simulink model "sub32_4n_model_run"  (R2023b)
settings: Solver=VariableStepAuto  StartTime=0.0  StopTime=5000E-12  FixedStep=1e-20  RelTol=1e-3
model workspace (MAT data in the model file):
  tp_delay = 1.25e-10
values from neighbouring files (symbols this model uses):
  tp_combinerA1_G8 = mean_CtoG + normrnd(0, stdev_CtoG)    [blockConf.m]
  tp_combinerA2_G4 = mean_CtoG + normrnd(0, stdev_CtoG)    [blockConf.m]
  tp_combinerA3_G2 = mean_CtoG + normrnd(0, stdev_CtoG)    [blockConf.m]
  tp_combinerA4_G1 = mean_CtoG + normrnd(0, stdev_CtoG)    [blockConf.m]
  tp_combinerB1_G8 = mean_CtoG + normrnd(0, stdev_CtoG)    [blockConf.m]
  tp_combinerB2_G4 = mean_CtoG + normrnd(0, stdev_CtoG)    [blockConf.m]
  tp_combinerB3_G2 = mean_CtoG + normrnd(0, stdev_CtoG)    [blockConf.m]
  tp_combinerB4_G1 = mean_CtoG + normrnd(0, stdev_CtoG)    [blockConf.m]
  tp_delay_1 = mean_DtoR + normrnd(0, stdev_DtoR)    [blockConf.m]
  tp_delay_10 = mean_DtoR + normrnd(0, stdev_DtoR)    [blockConf.m]
  tp_delay_11 = mean_DtoR + normrnd(0, stdev_DtoR)    [blockConf.m]
  tp_delay_12 = mean_DtoR + normrnd(0, stdev_DtoR)    [blockConf.m]
  tp_delay_13 = mean_DtoR + normrnd(0, stdev_DtoR)    [blockConf.m]
  tp_delay_14 = mean_DtoR + normrnd(0, stdev_DtoR)    [blockConf.m]
  tp_delay_15 = mean_DtoR + normrnd(0, stdev_DtoR)    [blockConf.m]
  tp_delay_16 = mean_DtoR + normrnd(0, stdev_DtoR)    [blockConf.m]
  tp_delay_17 = mean_DtoR + normrnd(0, stdev_DtoR)    [blockConf.m]
  tp_delay_18 = mean_DtoR + normrnd(0, stdev_DtoR)    [blockConf.m]
  tp_delay_19 = mean_DtoR + normrnd(0, stdev_DtoR)    [blockConf.m]
  tp_delay_2 = mean_DtoR + normrnd(0, stdev_DtoR)    [blockConf.m]
  tp_delay_20 = mean_DtoR + normrnd(0, stdev_DtoR)    [blockConf.m]
  tp_delay_21 = mean_DtoR + normrnd(0, stdev_DtoR)    [blockConf.m]
  tp_delay_22 = mean_DtoR + normrnd(0, stdev_DtoR)    [blockConf.m]
  tp_delay_23 = mean_DtoR + normrnd(0, stdev_DtoR)    [blockConf.m]
  tp_delay_24 = mean_DtoR + normrnd(0, stdev_DtoR)    [blockConf.m]
  tp_delay_25 = mean_DtoR + normrnd(0, stdev_DtoR)    [blockConf.m]
  tp_delay_26 = mean_DtoR + normrnd(0, stdev_DtoR)    [blockConf.m]
  tp_delay_27 = mean_DtoR + normrnd(0, stdev_DtoR)    [blockConf.m]
  tp_delay_28 = mean_DtoR + normrnd(0, stdev_DtoR)    [blockConf.m]
  tp_delay_29 = mean_DtoR + normrnd(0, stdev_DtoR)    [blockConf.m]
  tp_delay_3 = mean_DtoR + normrnd(0, stdev_DtoR)    [blockConf.m]
  tp_delay_30 = mean_DtoR + normrnd(0, stdev_DtoR)    [blockConf.m]
  tp_delay_31 = mean_DtoR + normrnd(0, stdev_DtoR)    [blockConf.m]
  tp_delay_32 = mean_DtoR + normrnd(0, stdev_DtoR)    [blockConf.m]
  tp_delay_4 = mean_DtoR + normrnd(0, stdev_DtoR)    [blockConf.m]
  tp_delay_5 = mean_DtoR + normrnd(0, stdev_DtoR)    [blockConf.m]
  tp_delay_6 = mean_DtoR + normrnd(0, stdev_DtoR)    [blockConf.m]
  tp_delay_7 = mean_DtoR + normrnd(0, stdev_DtoR)    [blockConf.m]
  tp_delay_8 = mean_DtoR + normrnd(0, stdev_DtoR)    [blockConf.m]
  tp_delay_9 = mean_DtoR + normrnd(0, stdev_DtoR)    [blockConf.m]
  tp_delay_b1 = mean_delay + normrnd(0, stdev_delay)    [blockConf.m]
  tp_delay_b10 = mean_delay + normrnd(0, stdev_delay)    [blockConf.m]
  tp_delay_b11 = mean_delay + normrnd(0, stdev_delay)    [blockConf.m]
  tp_delay_b12 = mean_delay + normrnd(0, stdev_delay)    [blockConf.m]
  tp_delay_b13 = mean_delay + normrnd(0, stdev_delay)    [blockConf.m]
  tp_delay_b14 = mean_delay + normrnd(0, stdev_delay)    [blockConf.m]
  tp_delay_b15 = mean_delay + normrnd(0, stdev_delay)    [blockConf.m]
  tp_delay_b16 = mean_delay + normrnd(0, stdev_delay)    [blockConf.m]
  tp_delay_b17 = mean_delay + normrnd(0, stdev_delay)    [blockConf.m]
  tp_delay_b18 = mean_delay + normrnd(0, stdev_delay)    [blockConf.m]
  tp_delay_b19 = mean_delay + normrnd(0, stdev_delay)    [blockConf.m]
  tp_delay_b2 = mean_delay + normrnd(0, stdev_delay)    [blockConf.m]
  tp_delay_b20 = mean_delay + normrnd(0, stdev_delay)    [blockConf.m]
  tp_delay_b21 = mean_delay + normrnd(0, stdev_delay)    [blockConf.m]
  tp_delay_b22 = mean_delay + normrnd(0, stdev_delay)    [blockConf.m]
  tp_delay_b23 = mean_delay + normrnd(0, stdev_delay)    [blockConf.m]
  tp_delay_b24 = mean_delay + normrnd(0, stdev_delay)    [blockConf.m]
  tp_delay_b25 = mean_delay + normrnd(0, stdev_delay)    [blockConf.m]
  tp_delay_b26 = mean_delay + normrnd(0, stdev_delay)    [blockConf.m]
  tp_delay_b27 = mean_delay + normrnd(0, stdev_delay)    [blockConf.m]
  tp_delay_b28 = mean_delay + normrnd(0, stdev_delay)    [blockConf.m]
  tp_delay_b29 = mean_delay + normrnd(0, stdev_delay)    [blockConf.m]
  tp_delay_b3 = mean_delay + normrnd(0, stdev_delay)    [blockConf.m]
  tp_delay_b30 = mean_delay + normrnd(0, stdev_delay)    [blockConf.m]
  tp_delay_b31 = mean_delay + normrnd(0, stdev_delay)    [blockConf.m]
  tp_delay_b4 = mean_delay + normrnd(0, stdev_delay)    [blockConf.m]
  tp_delay_b5 = mean_delay + normrnd(0, stdev_delay)    [blockConf.m]
  tp_delay_b6 = mean_delay + normrnd(0, stdev_delay)    [blockConf.m]
  tp_delay_b7 = mean_delay + normrnd(0, stdev_delay)    [blockConf.m]
  tp_delay_b8 = mean_delay + normrnd(0, stdev_delay)    [blockConf.m]
  tp_delay_b9 = mean_delay + normrnd(0, stdev_delay)    [blockConf.m]
  tp_pa_1 = mean_GtoP + normrnd(0, stdev_GtoP1)    [blockConf.m]
  tp_pa_2 = mean_GtoP + normrnd(0, stdev_GtoP2)    [blockConf.m]
  tp_pa_3 = mean_GtoP + normrnd(0, stdev_GtoP3)    [blockConf.m]
  tp_pa_4 = mean_GtoP + normrnd(0, stdev_GtoP4)    [blockConf.m]
  tp_router10_1 = mean_RtoC + normrnd(0, stdev_RtoC)    [blockConf.m]
  tp_router10_2 = mean_RtoC + normrnd(0, stdev_RtoC)    [blockConf.m]
  tp_router10_4 = mean_RtoC + normrnd(0, stdev_RtoC)    [blockConf.m]
  tp_router10_8 = mean_RtoC + normrnd(0, stdev_RtoC)    [blockConf.m]
  tp_router11_1 = mean_RtoC + normrnd(0, stdev_RtoC)    [blockConf.m]
  tp_router11_2 = mean_RtoC + normrnd(0, stdev_RtoC)    [blockConf.m]
  tp_router11_4 = mean_RtoC + normrnd(0, stdev_RtoC)    [blockConf.m]
  tp_router11_8 = mean_RtoC + normrnd(0, stdev_RtoC)    [blockConf.m]
  tp_router12_1 = mean_RtoC + normrnd(0, stdev_RtoC)    [blockConf.m]
  tp_router12_2 = mean_RtoC + normrnd(0, stdev_RtoC)    [blockConf.m]
  tp_router12_4 = mean_RtoC + normrnd(0, stdev_RtoC)    [blockConf.m]
  tp_router12_8 = mean_RtoC + normrnd(0, stdev_RtoC)    [blockConf.m]
  tp_router13_1 = mean_RtoC + normrnd(0, stdev_RtoC)    [blockConf.m]
  tp_router13_2 = mean_RtoC + normrnd(0, stdev_RtoC)    [blockConf.m]
  tp_router13_4 = mean_RtoC + normrnd(0, stdev_RtoC)    [blockConf.m]
  tp_router13_8 = mean_RtoC + normrnd(0, stdev_RtoC)    [blockConf.m]
  tp_router14_1 = mean_RtoC + normrnd(0, stdev_RtoC)    [blockConf.m]
  tp_router14_2 = mean_RtoC + normrnd(0, stdev_RtoC)    [blockConf.m]
  tp_router14_4 = mean_RtoC + normrnd(0, stdev_RtoC)    [blockConf.m]
  tp_router14_8 = mean_RtoC + normrnd(0, stdev_RtoC)    [blockConf.m]
  tp_router15_1 = mean_RtoC + normrnd(0, stdev_RtoC)    [blockConf.m]
  tp_router15_2 = mean_RtoC + normrnd(0, stdev_RtoC)    [blockConf.m]
  tp_router15_4 = mean_RtoC + normrnd(0, stdev_RtoC)    [blockConf.m]
  tp_router15_8 = mean_RtoC + normrnd(0, stdev_RtoC)    [blockConf.m]
  tp_router16_1 = mean_RtoC + normrnd(0, stdev_RtoC)    [blockConf.m]
  tp_router16_2 = mean_RtoC + normrnd(0, stdev_RtoC)    [blockConf.m]
  tp_router16_4 = mean_RtoC + normrnd(0, stdev_RtoC)    [blockConf.m]
  tp_router16_8 = mean_RtoC + normrnd(0, stdev_RtoC)    [blockConf.m]
  tp_router17_1 = mean_RtoC + normrnd(0, stdev_RtoC)    [blockConf.m]
  tp_router17_2 = mean_RtoC + normrnd(0, stdev_RtoC)    [blockConf.m]
  tp_router17_4 = mean_RtoC + normrnd(0, stdev_RtoC)    [blockConf.m]
  tp_router17_8 = mean_RtoC + normrnd(0, stdev_RtoC)    [blockConf.m]
  tp_router18_1 = mean_RtoC + normrnd(0, stdev_RtoC)    [blockConf.m]
  tp_router18_2 = mean_RtoC + normrnd(0, stdev_RtoC)    [blockConf.m]
  tp_router18_4 = mean_RtoC + normrnd(0, stdev_RtoC)    [blockConf.m]
  tp_router18_8 = mean_RtoC + normrnd(0, stdev_RtoC)    [blockConf.m]
  tp_router19_1 = mean_RtoC + normrnd(0, stdev_RtoC)    [blockConf.m]
  tp_router19_2 = mean_RtoC + normrnd(0, stdev_RtoC)    [blockConf.m]
  tp_router19_4 = mean_RtoC + normrnd(0, stdev_RtoC)    [blockConf.m]
  tp_router19_8 = mean_RtoC + normrnd(0, stdev_RtoC)    [blockConf.m]
  tp_router1_1 = mean_RtoC + normrnd(0, stdev_RtoC)    [blockConf.m]
  tp_router1_2 = mean_RtoC + normrnd(0, stdev_RtoC)    [blockConf.m]
  tp_router1_4 = mean_RtoC + normrnd(0, stdev_RtoC)    [blockConf.m]
  tp_router1_8 = mean_RtoC + normrnd(0, stdev_RtoC)    [blockConf.m]
  tp_router20_1 = mean_RtoC + normrnd(0, stdev_RtoC)    [blockConf.m]
  ... (+83 more)
undefined symbols (not defined in the file or in its folder): r10_1, r10_2, r10_4, r10_8, r11_1, r11_2, r11_4, r11_8, r12_1, r12_2, r12_4, r12_8, r13_1, r13_2, r13_4, r13_8, r14_1, r14_2, r14_4, r14_8, r15_1, r15_2, r15_4, r15_8, r16_1, r16_2, r16_4, r16_8, r1_1, r1_2, r1_4, r1_8, r2_1, r2_2, r2_4, r2_8, r3_1, r3_2, r3_4, r3_8, r4_1, r4_2, r4_4, r4_8, r5_1, r5_2, r5_4, r5_8, r6_1, r6_2, r6_4, r6_8, r7_1, r7_2, r7_4, r7_8, r8_1, r8_2, r8_4, r8_8 ... (+4)
libraries: fl_lib x15, nesl_utility x3, simulink x2
(part 1 of 2)
settings Model: PacingRate=0.010000  Creator=emman  LastModifiedBy=emman
settings SolverCC: EnableFixedStepZeroCrossing=on
settings OptimizationCC: ReuseModelBlockBuffer=off
settings DebuggingCC: SigSpecEnsureSampleTimeMsg=none

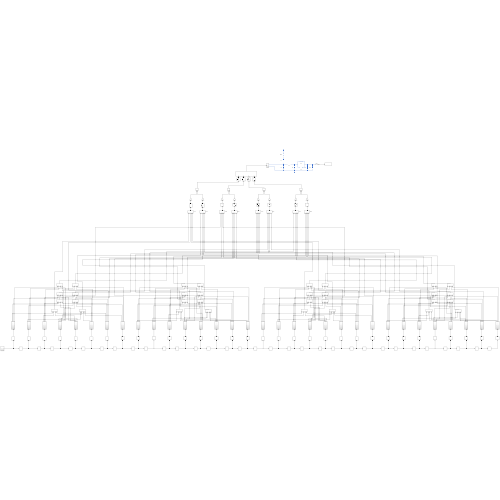
[thumbnail: Simulink's stored preview of the top-level diagram]
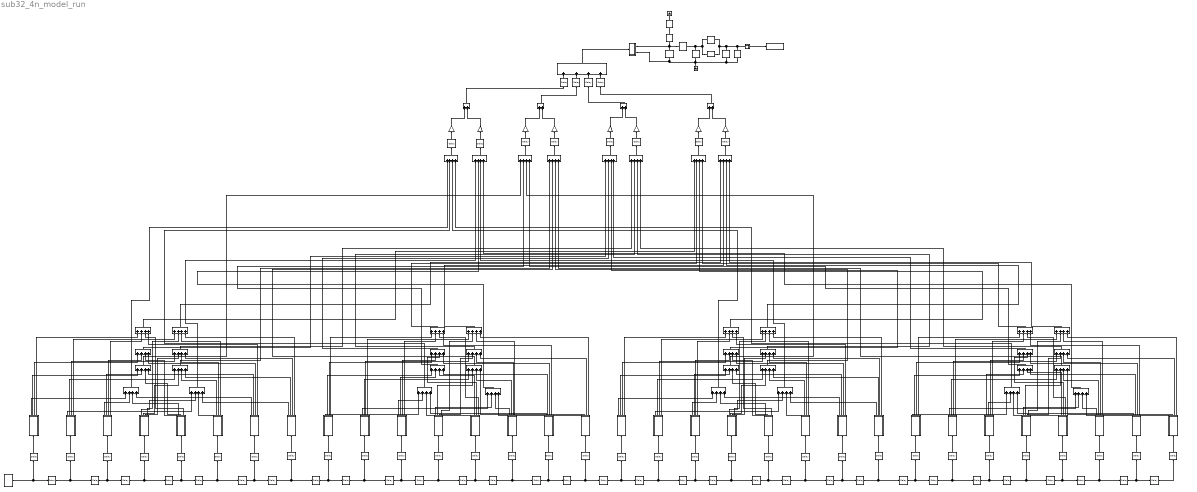
== system sub32_4n_model_run ==
  A<1> : Sum  Inputs=++++
  A<2> : Sum  Inputs=++++
  A<3> : Sum  Inputs=++++
  A<4> : Sum  Inputs=++++
  Add{,1..15,20..36} (33 alike) : Sum  Inputs=++++
  Add{16..19} (4 alike) : Sum
  B<1> : Sum  Inputs=++++
  B<2> : Sum  Inputs=++++
  B<3> : Sum  Inputs=++++
  B<4> : Sum  Inputs=++++
  C1 : fl_lib/Electrical/Electrical Elements/Capacitor  c=870e-15 F  r=0 Ohm  g=0 1/Ohm  i_specify=off  i_priority=None  i=0 A  i_nominal_specify=off  i_nominal_unit=A  i_nominal_value=1  v_specify=off  v_priority=None  v=0 V  v_nominal_specify=off  v_nominal_unit=V  v_nominal_value=1  vc_specify=off  vc_priority=High  vc=0 V  vc_nominal_specify=off  vc_nominal_unit=V  vc_nominal_value=1
  C2 : fl_lib/Electrical/Electrical Elements/Capacitor  c=1.1e-12 F  r=0 Ohm  g=0 1/Ohm  i_specify=off  i_priority=None  i=0 A  i_nominal_specify=off  i_nominal_unit=A  i_nominal_value=1  v_specify=off  v_priority=None  v=0 V  v_nominal_specify=off  v_nominal_unit=V  v_nominal_value=1  vc_specify=off  vc_priority=High  vc=0 V  vc_nominal_specify=off  vc_nominal_unit=V  vc_nominal_value=1
  C3 : fl_lib/Electrical/Electrical Elements/Capacitor  c=150e-15 F  r=0 Ohm  g=0 1/Ohm  i_specify=off  i_priority=None  i=0 A  i_nominal_specify=off  i_nominal_unit=A  i_nominal_value=1  v_specify=off  v_priority=None  v=0 V  v_nominal_specify=off  v_nominal_unit=V  v_nominal_value=1  vc_specify=off  vc_priority=High  vc=0 V  vc_nominal_specify=off  vc_nominal_unit=V  vc_nominal_value=1
  C4 : fl_lib/Electrical/Electrical Elements/Capacitor  c=70e-15 F  r=0 Ohm  g=0 1/Ohm  i_specify=off  i_priority=None  i=0 A  i_nominal_specify=off  i_nominal_unit=A  i_nominal_value=1  v_specify=off  v_priority=None  v=0 V  v_nominal_specify=off  v_nominal_unit=V  v_nominal_value=1  vc_specify=off  vc_priority=High  vc=0 V  vc_nominal_specify=off  vc_nominal_unit=V  vc_nominal_value=1
  C5 : fl_lib/Electrical/Electrical Elements/Capacitor  c=410e-15 F  r=0 Ohm  g=0 1/Ohm  i_specify=off  i_priority=None  i=0 A  i_nominal_specify=off  i_nominal_unit=A  i_nominal_value=1  v_specify=off  v_priority=None  v=0 V  v_nominal_specify=off  v_nominal_unit=V  v_nominal_value=1  vc_specify=off  vc_priority=High  vc=0 V  vc_nominal_specify=off  vc_nominal_unit=V  vc_nominal_value=1
  Current Source : Subsystem
  Electrical Reference : fl_lib/Electrical/Electrical Elements/Electrical Reference
  Electrical Reference1 : fl_lib/Electrical/Electrical Elements/Electrical Reference
  Gain : Gain  Gain=8
  Gain1 : Gain  Gain=8
  Gain2 : Gain  Gain=4
  Gain3 : Gain  Gain=4
  Gain4 : Gain  Gain=2
  Gain5 : Gain  Gain=2
  Gain6 : Gain
  Gain7 : Gain
  L1 : fl_lib/Electrical/Electrical Elements/Inductor  l=420e-12 H  r=0 Ohm  g=0 1/Ohm  i_specify=off  i_priority=None  i=0 A  i_nominal_specify=off  i_nominal_unit=A  i_nominal_value=1  v_specify=off  v_priority=None  v=0 V  v_nominal_specify=off  v_nominal_unit=V  v_nominal_value=1  i_L_specify=off  i_L_priority=High  i_L=0 A  i_L_nominal_specify=off  i_L_nominal_unit=A  i_L_nominal_value=1
  L2 : fl_lib/Electrical/Electrical Elements/Inductor  l=820e-12 H  r=0 Ohm  g=0 1/Ohm  i_specify=off  i_priority=None  i=0 A  i_nominal_specify=off  i_nominal_unit=A  i_nominal_value=1  v_specify=off  v_priority=None  v=0 V  v_nominal_specify=off  v_nominal_unit=V  v_nominal_value=1  i_L_specify=off  i_L_priority=High  i_L=0 A  i_L_nominal_specify=off  i_L_nominal_unit=A  i_L_nominal_value=1
  R0 : fl_lib/Electrical/Electrical Elements/Resistor  R=50 Ohm  i_specify=off  i_priority=None  i=0 A  i_nominal_specify=off  i_nominal_unit=A  i_nominal_value=1  v_specify=off  v_priority=None  v=0 V  v_nominal_specify=off  v_nominal_unit=V  v_nominal_value=1
  Simscape : Subsystem
      mask Display: disp('V')
  Subsystem : Subsystem
  Subsystem1 : Subsystem
  Subsystem10 : Subsystem
  Subsystem11 : Subsystem
  Subsystem12 : Subsystem
  Subsystem13 : Subsystem
  Subsystem14 : Subsystem
  Subsystem15 : Subsystem
  Subsystem16 : Subsystem
  Subsystem17 : Subsystem
  Subsystem18 : Subsystem
  Subsystem19 : Subsystem
  Subsystem2 : Subsystem
  Subsystem20 : Subsystem
  Subsystem21 : Subsystem
  Subsystem22 : Subsystem
  Subsystem23 : Subsystem
  Subsystem24 : Subsystem
  Subsystem25 : Subsystem
  Subsystem26 : Subsystem
  Subsystem27 : Subsystem
  Subsystem28 : Subsystem
  Subsystem29 : Subsystem
  Subsystem3 : Subsystem
  Subsystem30 : Subsystem
  Subsystem31 : Subsystem
  Subsystem32 : Subsystem
  Subsystem4 : Subsystem
  Subsystem5 : Subsystem
  Subsystem6 : Subsystem
  Subsystem7 : Subsystem
  Subsystem8 : Subsystem
  Subsystem9 : Subsystem
  To Workspace : ToWorkspace  VariableName=gpulse  SaveFormat=Timeseries  SampleTime=10e-12
  Transport Delay : TransportDelay  DelayTime=tp_delay_b1
  Transport Delay1 : TransportDelay  DelayTime=tp_delay_b2
  Transport Delay10 : TransportDelay  DelayTime=tp_delay_b11
  Transport Delay101 : TransportDelay  DelayTime=tp_delay_b22
  Transport Delay102 : TransportDelay  DelayTime=tp_delay_b23
  Transport Delay103 : TransportDelay  DelayTime=tp_delay_b24
  Transport Delay104 : TransportDelay  DelayTime=tp_delay_b25
  Transport Delay105 : TransportDelay  DelayTime=tp_delay_b26
  Transport Delay106 : TransportDelay  DelayTime=tp_delay_b16
  Transport Delay11 : TransportDelay  DelayTime=tp_delay_b12
  Transport Delay12 : TransportDelay  DelayTime=tp_delay_b13
  Transport Delay13 : TransportDelay  DelayTime=tp_delay_b14
  Transport Delay14 : TransportDelay  DelayTime=tp_delay_b15
  Transport Delay15 : TransportDelay  DelayTime=tp_delay_1
  Transport Delay16 : TransportDelay  DelayTime=tp_delay_2
  Transport Delay17 : TransportDelay  DelayTime=tp_delay_3
  Transport Delay18 : TransportDelay  DelayTime=tp_delay_4
  Transport Delay19 : TransportDelay  DelayTime=tp_delay_5
  Transport Delay2 : TransportDelay  DelayTime=tp_delay_b3
  Transport Delay20 : TransportDelay  DelayTime=tp_delay_6
  Transport Delay21 : TransportDelay  DelayTime=tp_delay_7
  Transport Delay22 : TransportDelay  DelayTime=tp_delay_8
  Transport Delay23 : TransportDelay  DelayTime=tp_delay_9
  Transport Delay24 : TransportDelay  DelayTime=tp_delay_10
  Transport Delay25 : TransportDelay  DelayTime=tp_delay_11
  Transport Delay26 : TransportDelay  DelayTime=tp_delay_12
  Transport Delay27 : TransportDelay  DelayTime=tp_delay_13
  Transport Delay28 : TransportDelay  DelayTime=tp_delay_14
  Transport Delay29 : TransportDelay  DelayTime=tp_delay_15
  Transport Delay3 : TransportDelay  DelayTime=tp_delay_b4
  Transport Delay30 : TransportDelay  DelayTime=tp_delay_16
  Transport Delay4 : TransportDelay  DelayTime=tp_delay_b5
  Transport Delay47 : TransportDelay  DelayTime=tp_combinerA1_G8
  Transport Delay48 : TransportDelay  DelayTime=tp_combinerB1_G8
  Transport Delay49 : TransportDelay  DelayTime=tp_combinerA2_G4
  Transport Delay5 : TransportDelay  DelayTime=tp_delay_b6
  Transport Delay50 : TransportDelay  DelayTime=tp_combinerB2_G4
  Transport Delay51 : TransportDelay  DelayTime=tp_combinerA3_G2
  Transport Delay52 : TransportDelay  DelayTime=tp_combinerB3_G2
  Transport Delay53 : TransportDelay  DelayTime=tp_combinerA4_G1
  Transport Delay54 : TransportDelay  DelayTime=tp_combinerB4_G1
  Transport Delay55 : TransportDelay  DelayTime=tp_pa_1  TransDelayFeedthrough=on
  Transport Delay56 : TransportDelay  DelayTime=tp_pa_2  TransDelayFeedthrough=on
  Transport Delay57 : TransportDelay  DelayTime=tp_pa_3  TransDelayFeedthrough=on
  Transport Delay58 : TransportDelay  DelayTime=tp_pa_4  TransDelayFeedthrough=on
  Transport Delay59 : TransportDelay  DelayTime=tp_delay_b17
  Transport Delay6 : TransportDelay  DelayTime=tp_delay_b7
  Transport Delay60 : TransportDelay  DelayTime=tp_delay_b18
  Transport Delay61 : TransportDelay  DelayTime=tp_delay_b27
  Transport Delay62 : TransportDelay  DelayTime=tp_delay_b28
  Transport Delay63 : TransportDelay  DelayTime=tp_delay_b29
  Transport Delay64 : TransportDelay  DelayTime=tp_delay_b30
  Transport Delay65 : TransportDelay  DelayTime=tp_delay_b31
  Transport Delay66 : TransportDelay  DelayTime=tp_delay_17
  Transport Delay67 : TransportDelay  DelayTime=tp_delay_18
  Transport Delay68 : TransportDelay  DelayTime=tp_delay_19
  Transport Delay69 : TransportDelay  DelayTime=tp_delay_20
  Transport Delay7 : TransportDelay  DelayTime=tp_delay_b8
  Transport Delay70 : TransportDelay  DelayTime=tp_delay_21
  Transport Delay71 : TransportDelay  DelayTime=tp_delay_b19
  Transport Delay72 : TransportDelay  DelayTime=tp_delay_22
  Transport Delay73 : TransportDelay  DelayTime=tp_delay_23
  Transport Delay74 : TransportDelay  DelayTime=tp_delay_24
  Transport Delay75 : TransportDelay  DelayTime=tp_delay_25
  Transport Delay76 : TransportDelay  DelayTime=tp_delay_26
  Transport Delay77 : TransportDelay  DelayTime=tp_delay_27
  Transport Delay78 : TransportDelay  DelayTime=tp_delay_28
  Transport Delay79 : TransportDelay  DelayTime=tp_delay_29
  Transport Delay8 : TransportDelay  DelayTime=tp_delay_b9
  Transport Delay80 : TransportDelay  DelayTime=tp_delay_30
  Transport Delay81 : TransportDelay  DelayTime=tp_delay_31
  Transport Delay82 : TransportDelay  DelayTime=tp_delay_b20
  Transport Delay83 : TransportDelay  DelayTime=tp_delay_32
  Transport Delay9 : TransportDelay  DelayTime=tp_delay_b10
  Transport Delay93 : TransportDelay  DelayTime=tp_delay_b21
  VDD : fl_lib/Electrical/Electrical Sources/DC Voltage Source  v0=0.8 V
  wires:
  Subsystem16/1(Out1) -> Add/1
  Subsystem18/1(Out1) -> Add/2
  Subsystem20/1(Out1) -> Add/3
  Subsystem17/1(Out1) -> Add1/1
  Subsystem21/1(Out1) -> Add1/3
  Subsystem23/1(Out1) -> Add1/4
  Subsystem19/1(Out1) -> Add1/2
  Subsystem16/2(Out2) -> Add2/1
  Subsystem20/2(Out2) -> Add2/3
  Subsystem22/2(Out2) -> Add2/4
  Subsystem18/2(Out2) -> Add2/2
  Subsystem17/2(Out2) -> Add3/1
  Subsystem19/2(Out2) -> Add3/2
  Subsystem21/2(Out2) -> Add3/3
  Subsystem23/2(Out2) -> Add3/4
  Subsystem17/3(Out3) -> Add5/1
  Subsystem22/3(Out3) -> Add4/4
  Subsystem16/4(Out4) -> Add6/1
  Subsystem19/3(Out3) -> Add5/2
  Subsystem20/4(Out4) -> Add6/3
  Subsystem18/4(Out4) -> Add6/2
  Subsystem21/4(Out4) -> Add7/3
  Subsystem18/3(Out3) -> Add4/2
  Subsystem16/3(Out3) -> Add4/1
  Subsystem23/4(Out4) -> Add7/4
  Subsystem19/4(Out4) -> Add7/2
  Subsystem20/3(Out3) -> Add4/3
  Subsystem17/4(Out4) -> Add7/1
  Subsystem21/3(Out3) -> Add5/3
  Subsystem23/3(Out3) -> Add5/4
  Subsystem8/4(Out4) -> Add14/1
  Subsystem3/4(Out4) -> Add15/3
  Subsystem5/2(Out2) -> Add11/2
  Subsystem2/2(Out2) -> Add10/4
  Subsystem7/1(Out1) -> Add9/1
  Subsystem5/1(Out1) -> Add9/2
  Subsystem4/1(Out1) -> Add8/3
  Subsystem1/4(Out4) -> Add15/4
  Subsystem8/3(Out3) -> Add12/1
  Subsystem2/3(Out3) -> Add12/4
  Subsystem7/3(Out3) -> Add13/1
  Subsystem4/3(Out3) -> Add12/3
  Subsystem4/2(Out2) -> Add10/3
  Subsystem3/2(Out2) -> Add11/3
  Subsystem1/3(Out3) -> Add13/4
  Subsystem6/3(Out3) -> Add12/2
  Subsystem1/1(Out1) -> Add9/4
  Subsystem7/4(Out4) -> Add15/1
  Subsystem2/1(Out1) -> Add8/4
  Subsystem8/2(Out2) -> Add10/1
  Subsystem2/4(Out4) -> Add14/4
  Subsystem6/4(Out4) -> Add14/2
  Subsystem1/2(Out2) -> Add11/4
  Subsystem8/1(Out1) -> Add8/1
  Subsystem3/3(Out3) -> Add13/3
  Subsystem7/2(Out2) -> Add11/1
  Subsystem4/4(Out4) -> Add14/3
  Subsystem5/4(Out4) -> Add15/2
  Subsystem3/1(Out1) -> Add9/3
  Subsystem5/3(Out3) -> Add13/2
  Gain/1 -> Add16/1
  Gain1/1 -> Add16/2
  Gain3/1 -> Add17/2
  Gain2/1 -> Add17/1
  Gain5/1 -> Add18/2
  Gain4/1 -> Add18/1
  Gain6/1 -> Add19/1
  Gain7/1 -> Add19/2
  Add16/1 -> Transport Delay55/1
  Add17/1 -> Transport Delay56/1
  Add18/1 -> Transport Delay57/1
  Add19/1 -> Transport Delay58/1
  Add20/1 -> Current Source/1(I)
  Simscape/1(Out) -> To Workspace/1  "output"
  Transport Delay3/1 -> Transport Delay4/1, Transport Delay19/1
  Transport Delay5/1 -> Transport Delay21/1, Transport Delay6/1
  Transport Delay4/1 -> Transport Delay20/1, Transport Delay5/1
  Transport Delay6/1 -> Transport Delay22/1, Transport Delay7/1
  Transport Delay13/1 -> Transport Delay29/1, Transport Delay14/1
  Transport Delay11/1 -> Transport Delay27/1, Transport Delay12/1
  Transport Delay10/1 -> Transport Delay26/1, Transport Delay11/1
  Transport Delay8/1 -> Transport Delay24/1, Transport Delay9/1
  Transport Delay9/1 -> Transport Delay25/1, Transport Delay10/1
  Transport Delay12/1 -> Transport Delay28/1, Transport Delay13/1
  A<3>/1 -> Transport Delay51/1
  A<4>/1 -> Transport Delay53/1
  B<4>/1 -> Transport Delay54/1
  B<3>/1 -> Transport Delay52/1
  Subsystem/1(Out1) -> Transport Delay15/1, Transport Delay/1
  Transport Delay/1 -> Transport Delay16/1, Transport Delay1/1
  Transport Delay1/1 -> Transport Delay17/1, Transport Delay2/1
  A<2>/1 -> Transport Delay49/1
  B<1>/1 -> Transport Delay48/1
  Transport Delay7/1 -> Transport Delay23/1, Transport Delay8/1
  Subsystem22/4(Out4) -> Add6/4
  Subsystem22/1(Out1) -> Add/4
  A<1>/1 -> Transport Delay47/1
  B<2>/1 -> Transport Delay50/1
  Transport Delay2/1 -> Transport Delay18/1, Transport Delay3/1
  Transport Delay15/1 -> Subsystem16/1(In1)
  Transport Delay16/1 -> Subsystem17/1(In1)
  Transport Delay17/1 -> Subsystem18/1(In1)
  Transport Delay18/1 -> Subsystem19/1(In1)
  Transport Delay19/1 -> Subsystem20/1(In1)
  Transport Delay20/1 -> Subsystem21/1(In1)
  Transport Delay21/1 -> Subsystem22/1(In1)
  Transport Delay22/1 -> Subsystem23/1(In1)
  Transport Delay23/1 -> Subsystem8/1(In1)
  Transport Delay24/1 -> Subsystem7/1(In1)
  Transport Delay25/1 -> Subsystem6/1(In1)
  Transport Delay26/1 -> Subsystem5/1(In1)
  Transport Delay27/1 -> Subsystem4/1(In1)
  Transport Delay28/1 -> Subsystem3/1(In1)
  Transport Delay29/1 -> Subsystem2/1(In1)
  Transport Delay30/1 -> Subsystem1/1(In1)
  Add/1 -> A<1>/1
  Add8/1 -> A<1>/2
  Add1/1 -> B<1>/1
  Add9/1 -> B<1>/2
  Add2/1 -> A<2>/1
  Add10/1 -> A<2>/2
  Add3/1 -> B<2>/1
  Add11/1 -> B<2>/2
  Add4/1 -> A<3>/1
  Add12/1 -> A<3>/2
  Add5/1 -> B<3>/1
  Add13/1 -> B<3>/2
  Add6/1 -> A<4>/1
  Add14/1 -> A<4>/2
  Add7/1 -> B<4>/1
  Add15/1 -> B<4>/2
  Transport Delay47/1 -> Gain/1
  Transport Delay48/1 -> Gain1/1
  Transport Delay49/1 -> Gain2/1
  Transport Delay50/1 -> Gain3/1
  Transport Delay51/1 -> Gain4/1
  Transport Delay52/1 -> Gain5/1
  Transport Delay53/1 -> Gain6/1
  Transport Delay54/1 -> Gain7/1
  Transport Delay55/1 -> Add20/1
  Transport Delay56/1 -> Add20/2
  Transport Delay57/1 -> Add20/3
  Transport Delay58/1 -> Add20/4
  Subsystem14/4(Out4) -> Add27/4
  Subsystem14/1(Out1) -> Add35/4
  Subsystem30/1(Out1) -> Add23/2
  Subsystem24/3(Out3) -> Add32/3
  Subsystem10/3(Out3) -> Add31/1
  Transport Delay66/1 -> Subsystem10/1(In1)
  Transport Delay103/1 -> Transport Delay75/1, Transport Delay104/1
  Transport Delay63/1 -> Transport Delay80/1, Transport Delay64/1
  Transport Delay60/1 -> Transport Delay68/1, Transport Delay71/1
  Subsystem28/3(Out3) -> Add25/3
  Subsystem12/3(Out3) -> Add31/2
  Transport Delay82/1 -> Transport Delay93/1, Transport Delay70/1
  Subsystem13/4(Out4) -> Add34/2
  Subsystem25/3(Out3) -> Add31/4
  Transport Delay105/1 -> Transport Delay77/1, Transport Delay61/1
  Subsystem29/2(Out2) -> Add24/2
  Transport Delay62/1 -> Transport Delay79/1, Transport Delay63/1
  Add36/1 -> B<1>/4
  Subsystem27/4(Out4) -> Add28/3
  Add28/1 -> B<4>/4
  Subsystem10/1(Out1) -> Add21/1
  Subsystem25/2(Out2) -> Add29/4
  Transport Delay104/1 -> Transport Delay76/1, Transport Delay105/1
  Subsystem25/1(Out1) -> Add21/4
  Subsystem11/2(Out2) -> Add30/1
  Subsystem12/2(Out2) -> Add29/2
  Subsystem15/2(Out2) -> Add29/3
  Subsystem26/2(Out2) -> Add30/4
  Transport Delay93/1 -> Transport Delay72/1, Transport Delay101/1
  Subsystem31/1(Out1) -> Add36/1
  Transport Delay76/1 -> Subsystem31/1(In1)
  Subsystem9/1(Out1) -> Add36/4
  Transport Delay77/1 -> Subsystem30/1(In1)
  Transport Delay75/1 -> Subsystem32/1(In1)
  Subsystem32/3(Out3) -> Add25/1
  Transport Delay80/1 -> Subsystem27/1(In1)
  Subsystem27/1(Out1) -> Add36/3
  Transport Delay72/1 -> Subsystem24/1(In1)
  Transport Delay69/1 -> Subsystem13/1(In1)
  Subsystem24/2(Out2) -> Add30/3
  Transport Delay67/1 -> Subsystem11/1(In1)
  Subsystem31/3(Out3) -> Add26/1
  Transport Delay14/1 -> Transport Delay106/1, Transport Delay30/1
  Subsystem11/4(Out4) -> Add34/1
  Subsystem29/4(Out4) -> Add28/2
  Subsystem24/1(Out1) -> Add22/3
  Transport Delay70/1 -> Subsystem15/1(In1)
  Transport Delay78/1 -> Subsystem29/1(In1)
  Add31/1 -> A<3>/3
  Subsystem15/3(Out3) -> Add31/3
  Transport Delay101/1 -> Transport Delay73/1, Transport Delay102/1
  Subsystem31/4(Out4) -> Add28/1
  Transport Delay102/1 -> Transport Delay74/1, Transport Delay103/1
  Subsystem28/2(Out2) -> Add23/3
  Add23/1 -> A<2>/4
  Subsystem10/4(Out4) -> Add33/1
  Subsystem15/4(Out4) -> Add33/3
  Transport Delay79/1 -> Subsystem28/1(In1)
  Subsystem9/4(Out4) -> Add28/4
  Transport Delay83/1 -> Subsystem9/1(In1)
  Subsystem14/2(Out2) -> Add23/4
  Transport Delay59/1 -> Transport Delay67/1, Transport Delay60/1
  Subsystem26/3(Out3) -> Add32/4
  Subsystem26/4(Out4) -> Add34/4
  Subsystem12/4(Out4) -> Add33/2
  Add26/1 -> B<3>/4
  Add27/1 -> A<4>/4
  Add24/1 -> B<2>/4
  Subsystem31/2(Out2) -> Add24/1
  Subsystem15/1(Out1) -> Add21/3
  Subsystem26/1(Out1) -> Add22/4
  Subsystem30/3(Out3) -> Add25/2
  Subsystem24/4(Out4) -> Add34/3
  Subsystem28/4(Out4) -> Add27/3
  Subsystem27/2(Out2) -> Add24/3
  Transport Delay68/1 -> Subsystem12/1(In1)
  Subsystem32/4(Out4) -> Add27/1
  Transport Delay64/1 -> Transport Delay81/1, Transport Delay65/1
  Subsystem13/2(Out2) -> Add30/2
  Subsystem29/1(Out1) -> Add36/2
  Transport Delay74/1 -> Subsystem26/1(In1)
  Subsystem13/3(Out3) -> Add32/2
  Subsystem14/3(Out3) -> Add25/4
  Transport Delay73/1 -> Subsystem25/1(In1)
  Subsystem30/4(Out4) -> Add27/2
  Subsystem9/2(Out2) -> Add24/4
  Subsystem32/2(Out2) -> Add23/1
  Subsystem32/1(Out1) -> Add35/1
  Subsystem30/2(Out2) -> Add35/2
  Subsystem10/2(Out2) -> Add29/1
  Subsystem9/3(Out3) -> Add26/4
  Subsystem28/1(Out1) -> Add35/3
  Subsystem27/3(Out3) -> Add26/3
  Subsystem12/1(Out1) -> Add21/2
  Transport Delay81/1 -> Subsystem14/1(In1)
  Add25/1 -> A<3>/4
  Subsystem11/3(Out3) -> Add32/1
  Add33/1 -> A<4>/3
  Subsystem13/1(Out1) -> Add22/2
  Transport Delay65/1 -> Transport Delay83/1
  Transport Delay61/1 -> Transport Delay78/1, Transport Delay62/1
  Transport Delay71/1 -> Transport Delay69/1, Transport Delay82/1
  Add21/1 -> A<1>/3
  Add32/1 -> B<3>/3
  Add35/1 -> A<1>/4
  Add22/1 -> B<1>/3
  Subsystem11/1(Out1) -> Add22/1
  Subsystem25/4(Out4) -> Add33/4
  Add29/1 -> A<2>/3
  Subsystem29/3(Out3) -> Add26/2
  Add30/1 -> B<2>/3
  Add34/1 -> B<4>/3
  Transport Delay106/1 -> Transport Delay59/1, Transport Delay66/1
  Subsystem6/1(Out1) -> Add8/2
  Subsystem6/2(Out2) -> Add10/2
  connections:
  Electrical Reference/LConn1 -- Current Source/RConn2 -- C1/RConn1 -- R0/RConn1 -- C5/RConn1 -- C3/RConn1
  C4/RConn1 -- L2/RConn1 -- Simscape/LConn1 -- R0/LConn1 -- C5/LConn1
  L2/LConn1 -- C4/LConn1 -- C3/LConn1 -- C2/RConn1
  VDD/RConn1 -- Electrical Reference1/LConn1
  L1/LConn1 -- VDD/LConn1
  C2/LConn1 -- Current Source/RConn1 -- L1/RConn1 -- C1/LConn1

== system sub32_4n_model_run/Current Source ==
  I : Inport
  Controlled Voltage Source : fl_lib/Electrical/Electrical Sources/Controlled Voltage Source
  Simulink-PS Converter : nesl_utility/Simulink-PS Converter  PhysicalDomain=network_engine_domain  SubClassName=ps_input  LeftPortType=input  RightPortType=output  PseudoPeriodic=off  Frequencies=[]  NoiseDistribution=none  NoiseParameters=[]  Unit=1  AffineConversion=off  FilteringAndDerivatives=zero  SimscapeFilterOrder=1  InputFilterTimeConstant=.001  UdotUserProvided=0
  Solver Configuration : nesl_utility/Solver Configuration  PhysicalDomain=network_engine_domain  SubClassName=solver  LeftPortType=input  RightPortType=generic  Tones=[]  Harmonics=[]  SimulateNoise=off  Profile=off  UseLocalSampling=off  EnableSwitchedLinearOptims=on  FrequencyDomain=off  UseCCode=off  RelTol=0.001  AbsTol=1e-06  MinStep=1e-09  ToWorkspace=off  RevertToSquareIcSolve=off  NumHomotopyIterations=100  PhasorMode=off  PhasorModeNumHarmonics=1  ConsistencySolver=NEWTON_FTOL  IndexReductionMethod=DerivativeReplacement  DoDC=on  ResidualTolerance=1e-15  ConsistencyTolSource=GLOBAL  ConsistencyAbsTol=0.001  ConsistencyRelTol=0.001  ConsistencyTolFactor=0.001  UseLocalSolver=off  LocalSolverChoice=NE_TRAPEZOIDAL_ADVANCER  ResolveIndetEquations=on  FunctionEvalNumThread=1  LocalSolverSampleTime=.001  DoFixedCost=on  MaxNonlinIter=3  MaxModeIter=2  ComputeImpulses=on  ImpulseIterations=2  LinearAlgebra=Full  LinearAlgebraNumThread=0  EquationFormulation=NE_TIME_EF  DelaysMemoryBudget=1024  AutomaticFiltering=off  FilteringTimeConstant=0.001  PartitionStorageMethod=AS_NEEDED  PartitionMemoryBudget=1024  PartitionMethod=FAST  MultibodyUseLocalSolver=off  MultibodyLocalSolverChoice=ODE1  MultibodyLocalSolverSampleTime=0.001
  Voltage-Controlled Current Source : fl_lib/Electrical/Electrical Sources/Voltage-Controlled Current Source  K=10 mS  v1_specify=off  v1_priority=None  v1=0 V  v1_nominal_specify=off  v1_nominal_unit=V  v1_nominal_value=1  i2_specify=off  i2_priority=None  i2=0 A  i2_nominal_specify=off  i2_nominal_unit=A  i2_nominal_value=1
      settings: InternalSimscapePortConfiguration="{\"Bottom\":[],\"Left\":[{\"id\":\"p1\",\"label\":\"+\",\"type\":\"foundation.electrical.electrical\"},{\"id\":\"head\",\"label\":\"\",\"type\":\"foundation.electrical.electrical\"}],\"Right\":[{\"id\":\"n1\",\"label\":\"-\",\"type\":\"foundation.electrical.electrical\"},{\"id\":\"tail\",\"label\":\"\",\"type\":\"foundation.electrical.electrical\"}],\"Top\":[]}"
  + : PMIOPort  Side=Right
  - : PMIOPort  Port=2  Side=Right
  wires:
  I/1 -> Simulink-PS Converter/1
  connections:
  Simulink-PS Converter/RConn1 -- Solver Configuration/RConn1 -- Controlled Voltage Source/RConn1
  -/RConn1 -- Controlled Voltage Source/RConn2 -- Voltage-Controlled Current Source/RConn1 -- Voltage-Controlled Current Source/RConn2
  +/RConn1 -- Voltage-Controlled Current Source/LConn2
  Controlled Voltage Source/LConn1 -- Voltage-Controlled Current Source/LConn1

== system sub32_4n_model_run/Simscape ==
  Electrical Reference1 : fl_lib/Electrical/Electrical Elements/Electrical Reference
  PS-S : nesl_utility/PS-Simulink Converter  PhysicalDomain=network_engine_domain  SubClassName=ps_output  LeftPortType=input  RightPortType=output  PseudoPeriodic=off  Frequencies=[]  VectorFormat=1-D array  Unit=V  AffineConversion=off
  Voltage Sensor : fl_lib/Electrical/Electrical Sensors/Voltage Sensor
  V : PMIOPort  Side=Left
  Out : Outport  VectorParamsAs1DForOutWhenUnconnected=off
  wires:
  PS-S/1 -> Out/1  "voltage"
  connections:
  PS-S/LConn1 -- Voltage Sensor/RConn1
  V/RConn1 -- Voltage Sensor/LConn1
  Electrical Reference1/LConn1 -- Voltage Sensor/RConn2

== system sub32_4n_model_run/Subsystem ==
  Add21 : Sum
  Ramp : simulink/Sources/Ramp  slope=80e+9  start=10e-12  InitialOutput=0
  Ramp1 : simulink/Sources/Ramp  slope=-80e+9  start=72.5e-12  InitialOutput=0
  Saturation : Saturate  UpperLimit=800e-3  LowerLimit=0
  Saturation1 : Saturate  UpperLimit=0  LowerLimit=-800e-3
  Out1 : Outport
  wires:
  Ramp/1 -> Saturation/1
  Saturation/1 -> Add21/1
  Ramp1/1 -> Saturation1/1
  Saturation1/1 -> Add21/2
  Add21/1 -> Out1/1

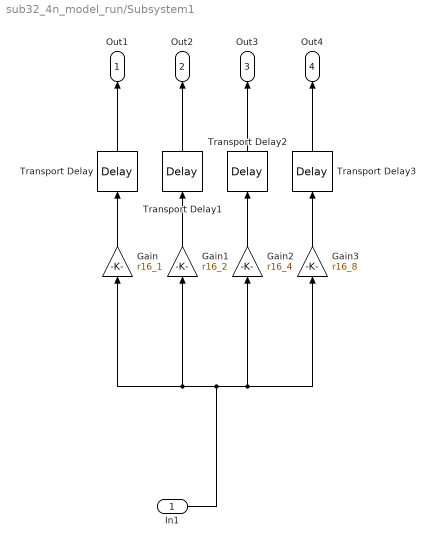
== system sub32_4n_model_run/Subsystem1 ==
  In1 : Inport
  Gain : Gain  Gain=r16_1
  Gain1 : Gain  Gain=r16_2
  Gain2 : Gain  Gain=r16_4
  Gain3 : Gain  Gain=r16_8
  Transport Delay : TransportDelay  DelayTime=tp_router16_1
  Transport Delay1 : TransportDelay  DelayTime=tp_router16_2
  Transport Delay2 : TransportDelay  DelayTime=tp_router16_4
  Transport Delay3 : TransportDelay  DelayTime=tp_router16_8
  Out1 : Outport
  Out2 : Outport  Port=2
  Out3 : Outport  Port=3
  Out4 : Outport  Port=4
  wires:
  Gain/1 -> Transport Delay/1
  Gain3/1 -> Transport Delay3/1
  Gain1/1 -> Transport Delay1/1
  In1/1 -> Gain1/1, Gain/1, Gain3/1, Gain2/1
  Gain2/1 -> Transport Delay2/1
  Transport Delay/1 -> Out1/1
  Transport Delay1/1 -> Out2/1
  Transport Delay2/1 -> Out3/1
  Transport Delay3/1 -> Out4/1

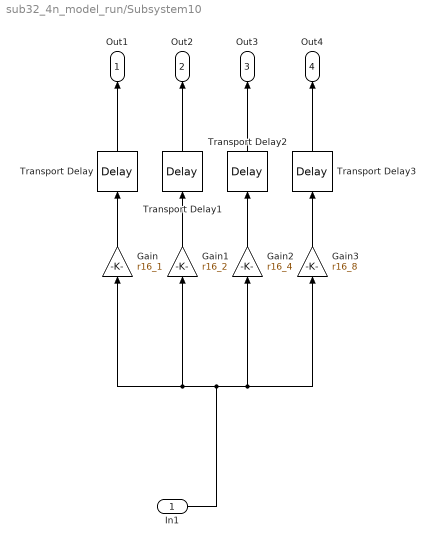
== system sub32_4n_model_run/Subsystem10 ==
  In1 : Inport
  Gain : Gain  Gain=r16_1
  Gain1 : Gain  Gain=r16_2
  Gain2 : Gain  Gain=r16_4
  Gain3 : Gain  Gain=r16_8
  Transport Delay : TransportDelay  DelayTime=tp_router17_1
  Transport Delay1 : TransportDelay  DelayTime=tp_router17_2
  Transport Delay2 : TransportDelay  DelayTime=tp_router17_4
  Transport Delay3 : TransportDelay  DelayTime=tp_router17_8
  Out1 : Outport
  Out2 : Outport  Port=2
  Out3 : Outport  Port=3
  Out4 : Outport  Port=4
  wires:
  Gain/1 -> Transport Delay/1
  Gain3/1 -> Transport Delay3/1
  Gain1/1 -> Transport Delay1/1
  In1/1 -> Gain1/1, Gain/1, Gain3/1, Gain2/1
  Gain2/1 -> Transport Delay2/1
  Transport Delay/1 -> Out1/1
  Transport Delay1/1 -> Out2/1
  Transport Delay2/1 -> Out3/1
  Transport Delay3/1 -> Out4/1

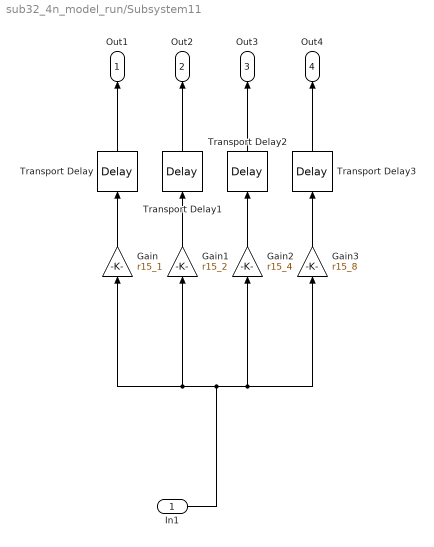
== system sub32_4n_model_run/Subsystem11 ==
  In1 : Inport
  Gain : Gain  Gain=r15_1
  Gain1 : Gain  Gain=r15_2
  Gain2 : Gain  Gain=r15_4
  Gain3 : Gain  Gain=r15_8
  Transport Delay : TransportDelay  DelayTime=tp_router18_1
  Transport Delay1 : TransportDelay  DelayTime=tp_router18_2
  Transport Delay2 : TransportDelay  DelayTime=tp_router18_4
  Transport Delay3 : TransportDelay  DelayTime=tp_router18_8
  Out1 : Outport
  Out2 : Outport  Port=2
  Out3 : Outport  Port=3
  Out4 : Outport  Port=4
  wires:
  Gain/1 -> Transport Delay/1
  Gain3/1 -> Transport Delay3/1
  Gain1/1 -> Transport Delay1/1
  In1/1 -> Gain1/1, Gain/1, Gain3/1, Gain2/1
  Gain2/1 -> Transport Delay2/1
  Transport Delay/1 -> Out1/1
  Transport Delay1/1 -> Out2/1
  Transport Delay2/1 -> Out3/1
  Transport Delay3/1 -> Out4/1

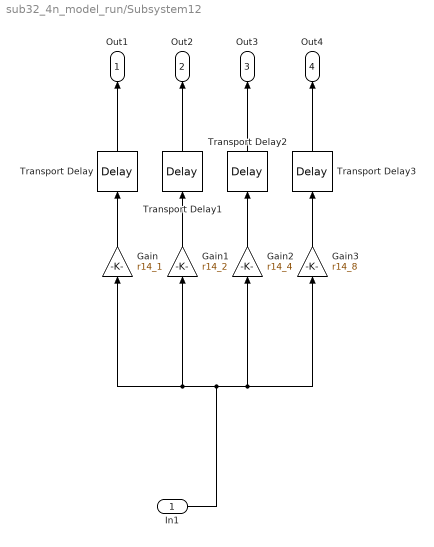
== system sub32_4n_model_run/Subsystem12 ==
  In1 : Inport
  Gain : Gain  Gain=r14_1
  Gain1 : Gain  Gain=r14_2
  Gain2 : Gain  Gain=r14_4
  Gain3 : Gain  Gain=r14_8
  Transport Delay : TransportDelay  DelayTime=tp_router19_1
  Transport Delay1 : TransportDelay  DelayTime=tp_router19_2
  Transport Delay2 : TransportDelay  DelayTime=tp_router19_4
  Transport Delay3 : TransportDelay  DelayTime=tp_router19_8
  Out1 : Outport
  Out2 : Outport  Port=2
  Out3 : Outport  Port=3
  Out4 : Outport  Port=4
  wires:
  Gain/1 -> Transport Delay/1
  Gain3/1 -> Transport Delay3/1
  Gain1/1 -> Transport Delay1/1
  In1/1 -> Gain1/1, Gain/1, Gain3/1, Gain2/1
  Gain2/1 -> Transport Delay2/1
  Transport Delay/1 -> Out1/1
  Transport Delay1/1 -> Out2/1
  Transport Delay2/1 -> Out3/1
  Transport Delay3/1 -> Out4/1

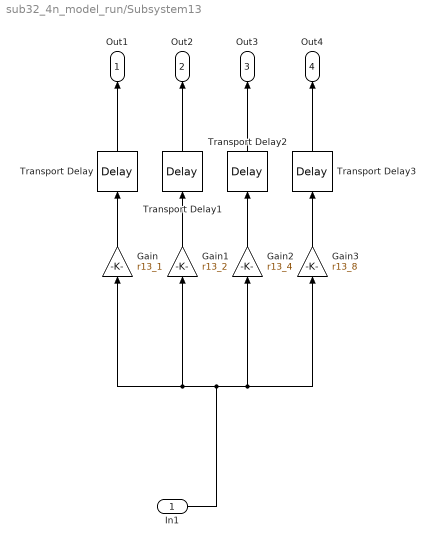
== system sub32_4n_model_run/Subsystem13 ==
  In1 : Inport
  Gain : Gain  Gain=r13_1
  Gain1 : Gain  Gain=r13_2
  Gain2 : Gain  Gain=r13_4
  Gain3 : Gain  Gain=r13_8
  Transport Delay : TransportDelay  DelayTime=tp_router20_1
  Transport Delay1 : TransportDelay  DelayTime=tp_router20_2
  Transport Delay2 : TransportDelay  DelayTime=tp_router20_4
  Transport Delay3 : TransportDelay  DelayTime=tp_router20_8
  Out1 : Outport
  Out2 : Outport  Port=2
  Out3 : Outport  Port=3
  Out4 : Outport  Port=4
  wires:
  Gain/1 -> Transport Delay/1
  Gain3/1 -> Transport Delay3/1
  Gain1/1 -> Transport Delay1/1
  In1/1 -> Gain1/1, Gain/1, Gain3/1, Gain2/1
  Gain2/1 -> Transport Delay2/1
  Transport Delay/1 -> Out1/1
  Transport Delay1/1 -> Out2/1
  Transport Delay2/1 -> Out3/1
  Transport Delay3/1 -> Out4/1

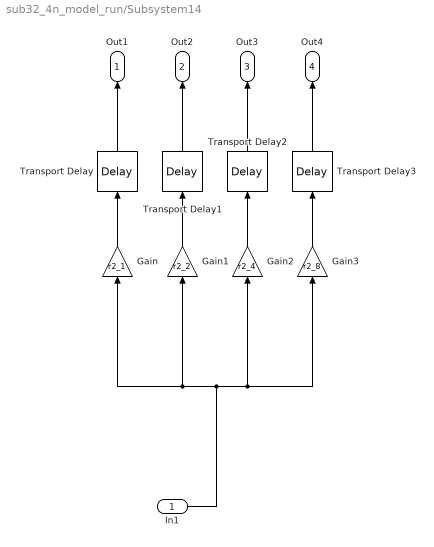
== system sub32_4n_model_run/Subsystem14 ==
  In1 : Inport
  Gain : Gain  Gain=r2_1
  Gain1 : Gain  Gain=r2_2
  Gain2 : Gain  Gain=r2_4
  Gain3 : Gain  Gain=r2_8
  Transport Delay : TransportDelay  DelayTime=tp_router31_1
  Transport Delay1 : TransportDelay  DelayTime=tp_router31_2
  Transport Delay2 : TransportDelay  DelayTime=tp_router31_4
  Transport Delay3 : TransportDelay  DelayTime=tp_router31_8
  Out1 : Outport
  Out2 : Outport  Port=2
  Out3 : Outport  Port=3
  Out4 : Outport  Port=4
  wires:
  Gain/1 -> Transport Delay/1
  Gain3/1 -> Transport Delay3/1
  Gain1/1 -> Transport Delay1/1
  In1/1 -> Gain1/1, Gain/1, Gain3/1, Gain2/1
  Gain2/1 -> Transport Delay2/1
  Transport Delay/1 -> Out1/1
  Transport Delay1/1 -> Out2/1
  Transport Delay2/1 -> Out3/1
  Transport Delay3/1 -> Out4/1

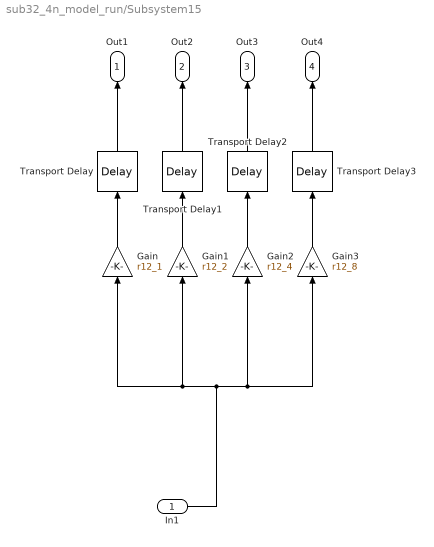
== system sub32_4n_model_run/Subsystem15 ==
  In1 : Inport
  Gain : Gain  Gain=r12_1
  Gain1 : Gain  Gain=r12_2
  Gain2 : Gain  Gain=r12_4
  Gain3 : Gain  Gain=r12_8
  Transport Delay : TransportDelay  DelayTime=tp_router21_1
  Transport Delay1 : TransportDelay  DelayTime=tp_router21_2
  Transport Delay2 : TransportDelay  DelayTime=tp_router21_4
  Transport Delay3 : TransportDelay  DelayTime=tp_router21_8
  Out1 : Outport
  Out2 : Outport  Port=2
  Out3 : Outport  Port=3
  Out4 : Outport  Port=4
  wires:
  Gain/1 -> Transport Delay/1
  Gain3/1 -> Transport Delay3/1
  Gain1/1 -> Transport Delay1/1
  In1/1 -> Gain1/1, Gain/1, Gain3/1, Gain2/1
  Gain2/1 -> Transport Delay2/1
  Transport Delay/1 -> Out1/1
  Transport Delay1/1 -> Out2/1
  Transport Delay2/1 -> Out3/1
  Transport Delay3/1 -> Out4/1

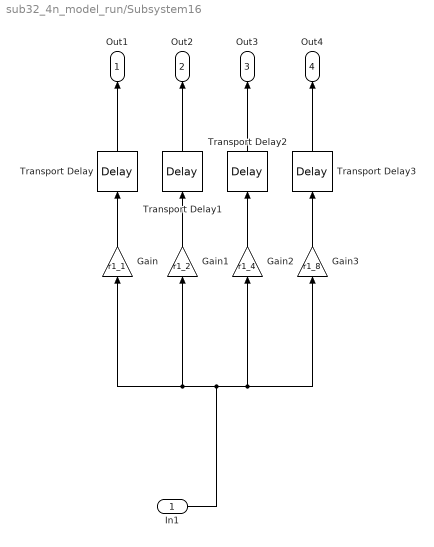
== system sub32_4n_model_run/Subsystem16 ==
  In1 : Inport
  Gain : Gain  Gain=r1_1
  Gain1 : Gain  Gain=r1_2
  Gain2 : Gain  Gain=r1_4
  Gain3 : Gain  Gain=r1_8
  Transport Delay : TransportDelay  DelayTime=tp_router1_1
  Transport Delay1 : TransportDelay  DelayTime=tp_router1_2
  Transport Delay2 : TransportDelay  DelayTime=tp_router1_4
  Transport Delay3 : TransportDelay  DelayTime=tp_router1_8
  Out1 : Outport
  Out2 : Outport  Port=2
  Out3 : Outport  Port=3
  Out4 : Outport  Port=4
  wires:
  Gain/1 -> Transport Delay/1
  Gain3/1 -> Transport Delay3/1
  Gain1/1 -> Transport Delay1/1
  In1/1 -> Gain1/1, Gain/1, Gain3/1, Gain2/1
  Gain2/1 -> Transport Delay2/1
  Transport Delay/1 -> Out1/1
  Transport Delay1/1 -> Out2/1
  Transport Delay2/1 -> Out3/1
  Transport Delay3/1 -> Out4/1

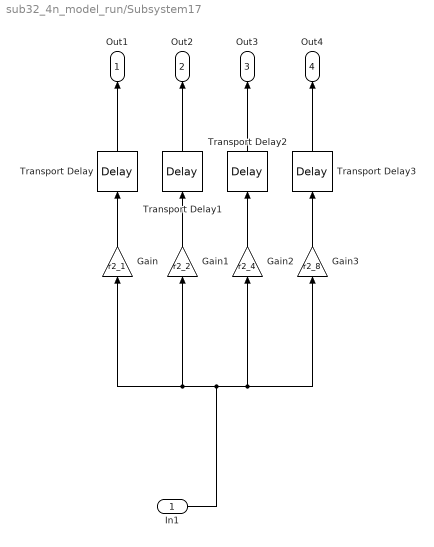
== system sub32_4n_model_run/Subsystem17 ==
  In1 : Inport
  Gain : Gain  Gain=r2_1
  Gain1 : Gain  Gain=r2_2
  Gain2 : Gain  Gain=r2_4
  Gain3 : Gain  Gain=r2_8
  Transport Delay : TransportDelay  DelayTime=tp_router2_1
  Transport Delay1 : TransportDelay  DelayTime=tp_router2_2
  Transport Delay2 : TransportDelay  DelayTime=tp_router2_4
  Transport Delay3 : TransportDelay  DelayTime=tp_router2_8
  Out1 : Outport
  Out2 : Outport  Port=2
  Out3 : Outport  Port=3
  Out4 : Outport  Port=4
  wires:
  Gain/1 -> Transport Delay/1
  Gain3/1 -> Transport Delay3/1
  Gain1/1 -> Transport Delay1/1
  In1/1 -> Gain1/1, Gain/1, Gain3/1, Gain2/1
  Gain2/1 -> Transport Delay2/1
  Transport Delay/1 -> Out1/1
  Transport Delay1/1 -> Out2/1
  Transport Delay2/1 -> Out3/1
  Transport Delay3/1 -> Out4/1

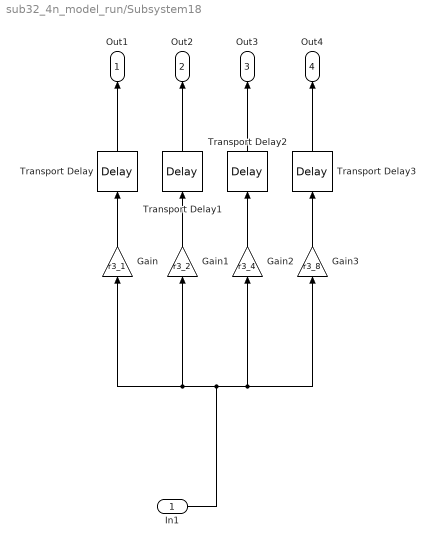
== system sub32_4n_model_run/Subsystem18 ==
  In1 : Inport
  Gain : Gain  Gain=r3_1
  Gain1 : Gain  Gain=r3_2
  Gain2 : Gain  Gain=r3_4
  Gain3 : Gain  Gain=r3_8
  Transport Delay : TransportDelay  DelayTime=tp_router3_1
  Transport Delay1 : TransportDelay  DelayTime=tp_router3_2
  Transport Delay2 : TransportDelay  DelayTime=tp_router3_4
  Transport Delay3 : TransportDelay  DelayTime=tp_router3_8
  Out1 : Outport
  Out2 : Outport  Port=2
  Out3 : Outport  Port=3
  Out4 : Outport  Port=4
  wires:
  Gain/1 -> Transport Delay/1
  Gain3/1 -> Transport Delay3/1
  Gain1/1 -> Transport Delay1/1
  In1/1 -> Gain1/1, Gain/1, Gain3/1, Gain2/1
  Gain2/1 -> Transport Delay2/1
  Transport Delay/1 -> Out1/1
  Transport Delay1/1 -> Out2/1
  Transport Delay2/1 -> Out3/1
  Transport Delay3/1 -> Out4/1

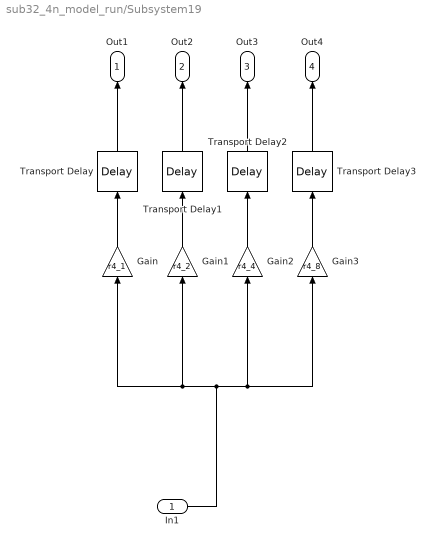
== system sub32_4n_model_run/Subsystem19 ==
  In1 : Inport
  Gain : Gain  Gain=r4_1
  Gain1 : Gain  Gain=r4_2
  Gain2 : Gain  Gain=r4_4
  Gain3 : Gain  Gain=r4_8
  Transport Delay : TransportDelay  DelayTime=tp_router4_1
  Transport Delay1 : TransportDelay  DelayTime=tp_router4_2
  Transport Delay2 : TransportDelay  DelayTime=tp_router4_4
  Transport Delay3 : TransportDelay  DelayTime=tp_router4_8
  Out1 : Outport
  Out2 : Outport  Port=2
  Out3 : Outport  Port=3
  Out4 : Outport  Port=4
  wires:
  Gain/1 -> Transport Delay/1
  Gain3/1 -> Transport Delay3/1
  Gain1/1 -> Transport Delay1/1
  In1/1 -> Gain1/1, Gain/1, Gain3/1, Gain2/1
  Gain2/1 -> Transport Delay2/1
  Transport Delay/1 -> Out1/1
  Transport Delay1/1 -> Out2/1
  Transport Delay2/1 -> Out3/1
  Transport Delay3/1 -> Out4/1

== system sub32_4n_model_run/Subsystem2 ==
  In1 : Inport
  Gain : Gain  Gain=r15_1
  Gain1 : Gain  Gain=r15_2
  Gain2 : Gain  Gain=r15_4
  Gain3 : Gain  Gain=r15_8
  Transport Delay : TransportDelay  DelayTime=tp_router15_1
  Transport Delay1 : TransportDelay  DelayTime=tp_router15_2
  Transport Delay2 : TransportDelay  DelayTime=tp_router15_4
  Transport Delay3 : TransportDelay  DelayTime=tp_router15_8
  Out1 : Outport
  Out2 : Outport  Port=2
  Out3 : Outport  Port=3
  Out4 : Outport  Port=4
  wires:
  Gain/1 -> Transport Delay/1
  Gain3/1 -> Transport Delay3/1
  Gain1/1 -> Transport Delay1/1
  In1/1 -> Gain1/1, Gain/1, Gain3/1, Gain2/1
  Gain2/1 -> Transport Delay2/1
  Transport Delay/1 -> Out1/1
  Transport Delay1/1 -> Out2/1
  Transport Delay2/1 -> Out3/1
  Transport Delay3/1 -> Out4/1

== system sub32_4n_model_run/Subsystem20 ==
  In1 : Inport
  Gain : Gain  Gain=r5_1
  Gain1 : Gain  Gain=r5_2
  Gain2 : Gain  Gain=r5_4
  Gain3 : Gain  Gain=r5_8
  Transport Delay : TransportDelay  DelayTime=tp_router5_1
  Transport Delay1 : TransportDelay  DelayTime=tp_router5_2
  Transport Delay2 : TransportDelay  DelayTime=tp_router5_4
  Transport Delay3 : TransportDelay  DelayTime=tp_router5_8
  Out1 : Outport
  Out2 : Outport  Port=2
  Out3 : Outport  Port=3
  Out4 : Outport  Port=4
  wires:
  Gain/1 -> Transport Delay/1
  Gain3/1 -> Transport Delay3/1
  Gain1/1 -> Transport Delay1/1
  In1/1 -> Gain1/1, Gain/1, Gain3/1, Gain2/1
  Gain2/1 -> Transport Delay2/1
  Transport Delay/1 -> Out1/1
  Transport Delay1/1 -> Out2/1
  Transport Delay2/1 -> Out3/1
  Transport Delay3/1 -> Out4/1

== system sub32_4n_model_run/Subsystem21 ==
  In1 : Inport
  Gain : Gain  Gain=r6_1
  Gain1 : Gain  Gain=r6_2
  Gain2 : Gain  Gain=r6_4
  Gain3 : Gain  Gain=r6_8
  Transport Delay : TransportDelay  DelayTime=tp_router6_1
  Transport Delay1 : TransportDelay  DelayTime=tp_router6_2
  Transport Delay2 : TransportDelay  DelayTime=tp_router6_4
  Transport Delay3 : TransportDelay  DelayTime=tp_router6_8
  Out1 : Outport
  Out2 : Outport  Port=2
  Out3 : Outport  Port=3
  Out4 : Outport  Port=4
  wires:
  Gain/1 -> Transport Delay/1
  Gain3/1 -> Transport Delay3/1
  Gain1/1 -> Transport Delay1/1
  In1/1 -> Gain1/1, Gain/1, Gain3/1, Gain2/1
  Gain2/1 -> Transport Delay2/1
  Transport Delay/1 -> Out1/1
  Transport Delay1/1 -> Out2/1
  Transport Delay2/1 -> Out3/1
  Transport Delay3/1 -> Out4/1

== system sub32_4n_model_run/Subsystem22 ==
  In1 : Inport
  Gain : Gain  Gain=r7_1
  Gain1 : Gain  Gain=r7_2
  Gain2 : Gain  Gain=r7_4
  Gain3 : Gain  Gain=r7_8
  Transport Delay : TransportDelay  DelayTime=tp_router7_1
  Transport Delay1 : TransportDelay  DelayTime=tp_router7_2
  Transport Delay2 : TransportDelay  DelayTime=tp_router7_4
  Transport Delay3 : TransportDelay  DelayTime=tp_router7_8
  Out1 : Outport
  Out2 : Outport  Port=2
  Out3 : Outport  Port=3
  Out4 : Outport  Port=4
  wires:
  Gain/1 -> Transport Delay/1
  Gain3/1 -> Transport Delay3/1
  Gain1/1 -> Transport Delay1/1
  In1/1 -> Gain1/1, Gain/1, Gain3/1, Gain2/1
  Gain2/1 -> Transport Delay2/1
  Transport Delay/1 -> Out1/1
  Transport Delay1/1 -> Out2/1
  Transport Delay2/1 -> Out3/1
  Transport Delay3/1 -> Out4/1

== system sub32_4n_model_run/Subsystem23 ==
  In1 : Inport
  Gain : Gain  Gain=r8_1
  Gain1 : Gain  Gain=r8_2
  Gain2 : Gain  Gain=r8_4
  Gain3 : Gain  Gain=r8_8
  Transport Delay : TransportDelay  DelayTime=tp_router8_1
  Transport Delay1 : TransportDelay  DelayTime=tp_router8_2
  Transport Delay2 : TransportDelay  DelayTime=tp_router8_4
  Transport Delay3 : TransportDelay  DelayTime=tp_router8_8
  Out1 : Outport
  Out2 : Outport  Port=2
  Out3 : Outport  Port=3
  Out4 : Outport  Port=4
  wires:
  Gain/1 -> Transport Delay/1
  Gain3/1 -> Transport Delay3/1
  Gain1/1 -> Transport Delay1/1
  In1/1 -> Gain1/1, Gain/1, Gain3/1, Gain2/1
  Gain2/1 -> Transport Delay2/1
  Transport Delay/1 -> Out1/1
  Transport Delay1/1 -> Out2/1
  Transport Delay2/1 -> Out3/1
  Transport Delay3/1 -> Out4/1

== system sub32_4n_model_run/Subsystem24 ==
  In1 : Inport
  Gain : Gain  Gain=r11_1
  Gain1 : Gain  Gain=r11_2
  Gain2 : Gain  Gain=r11_4
  Gain3 : Gain  Gain=r11_8
  Transport Delay : TransportDelay  DelayTime=tp_router22_1
  Transport Delay1 : TransportDelay  DelayTime=tp_router22_2
  Transport Delay2 : TransportDelay  DelayTime=tp_router22_4
  Transport Delay3 : TransportDelay  DelayTime=tp_router22_8
  Out1 : Outport
  Out2 : Outport  Port=2
  Out3 : Outport  Port=3
  Out4 : Outport  Port=4
  wires:
  Gain/1 -> Transport Delay/1
  Gain3/1 -> Transport Delay3/1
  Gain1/1 -> Transport Delay1/1
  In1/1 -> Gain1/1, Gain/1, Gain3/1, Gain2/1
  Gain2/1 -> Transport Delay2/1
  Transport Delay/1 -> Out1/1
  Transport Delay1/1 -> Out2/1
  Transport Delay2/1 -> Out3/1
  Transport Delay3/1 -> Out4/1

== system sub32_4n_model_run/Subsystem25 ==
  In1 : Inport
  Gain : Gain  Gain=r10_1
  Gain1 : Gain  Gain=r10_2
  Gain2 : Gain  Gain=r10_4
  Gain3 : Gain  Gain=r10_8
  Transport Delay : TransportDelay  DelayTime=tp_router23_1
  Transport Delay1 : TransportDelay  DelayTime=tp_router23_2
  Transport Delay2 : TransportDelay  DelayTime=tp_router23_4
  Transport Delay3 : TransportDelay  DelayTime=tp_router23_8
  Out1 : Outport
  Out2 : Outport  Port=2
  Out3 : Outport  Port=3
  Out4 : Outport  Port=4
  wires:
  Gain/1 -> Transport Delay/1
  Gain3/1 -> Transport Delay3/1
  Gain1/1 -> Transport Delay1/1
  In1/1 -> Gain1/1, Gain/1, Gain3/1, Gain2/1
  Gain2/1 -> Transport Delay2/1
  Transport Delay/1 -> Out1/1
  Transport Delay1/1 -> Out2/1
  Transport Delay2/1 -> Out3/1
  Transport Delay3/1 -> Out4/1

== system sub32_4n_model_run/Subsystem26 ==
  In1 : Inport
  Gain : Gain  Gain=r9_1
  Gain1 : Gain  Gain=r9_2
  Gain2 : Gain  Gain=r9_4
  Gain3 : Gain  Gain=r9_8
  Transport Delay : TransportDelay  DelayTime=tp_router24_1
  Transport Delay1 : TransportDelay  DelayTime=tp_router24_2
  Transport Delay2 : TransportDelay  DelayTime=tp_router24_4
  Transport Delay3 : TransportDelay  DelayTime=tp_router24_8
  Out1 : Outport
  Out2 : Outport  Port=2
  Out3 : Outport  Port=3
  Out4 : Outport  Port=4
  wires:
  Gain/1 -> Transport Delay/1
  Gain3/1 -> Transport Delay3/1
  Gain1/1 -> Transport Delay1/1
  In1/1 -> Gain1/1, Gain/1, Gain3/1, Gain2/1
  Gain2/1 -> Transport Delay2/1
  Transport Delay/1 -> Out1/1
  Transport Delay1/1 -> Out2/1
  Transport Delay2/1 -> Out3/1
  Transport Delay3/1 -> Out4/1

== system sub32_4n_model_run/Subsystem27 ==
  In1 : Inport
  Gain : Gain  Gain=r3_1
  Gain1 : Gain  Gain=r3_2
  Gain2 : Gain  Gain=r3_4
  Gain3 : Gain  Gain=r3_8
  Transport Delay : TransportDelay  DelayTime=tp_router30_1
  Transport Delay1 : TransportDelay  DelayTime=tp_router30_2
  Transport Delay2 : TransportDelay  DelayTime=tp_router30_4
  Transport Delay3 : TransportDelay  DelayTime=tp_router30_8
  Out1 : Outport
  Out2 : Outport  Port=2
  Out3 : Outport  Port=3
  Out4 : Outport  Port=4
  wires:
  Gain/1 -> Transport Delay/1
  Gain3/1 -> Transport Delay3/1
  Gain1/1 -> Transport Delay1/1
  In1/1 -> Gain1/1, Gain/1, Gain3/1, Gain2/1
  Gain2/1 -> Transport Delay2/1
  Transport Delay/1 -> Out1/1
  Transport Delay1/1 -> Out2/1
  Transport Delay2/1 -> Out3/1
  Transport Delay3/1 -> Out4/1

== system sub32_4n_model_run/Subsystem28 ==
  In1 : Inport
  Gain : Gain  Gain=r4_1
  Gain1 : Gain  Gain=r4_2
  Gain2 : Gain  Gain=r4_4
  Gain3 : Gain  Gain=r4_8
  Transport Delay : TransportDelay  DelayTime=tp_router29_1
  Transport Delay1 : TransportDelay  DelayTime=tp_router29_2
  Transport Delay2 : TransportDelay  DelayTime=tp_router29_4
  Transport Delay3 : TransportDelay  DelayTime=tp_router29_8
  Out1 : Outport
  Out2 : Outport  Port=2
  Out3 : Outport  Port=3
  Out4 : Outport  Port=4
  wires:
  Gain/1 -> Transport Delay/1
  Gain3/1 -> Transport Delay3/1
  Gain1/1 -> Transport Delay1/1
  In1/1 -> Gain1/1, Gain/1, Gain3/1, Gain2/1
  Gain2/1 -> Transport Delay2/1
  Transport Delay/1 -> Out1/1
  Transport Delay1/1 -> Out2/1
  Transport Delay2/1 -> Out3/1
  Transport Delay3/1 -> Out4/1
